simulink model "chap7_1sim"  (R2019a)
settings: Solver=ode45  StartTime=0.0  StopTime=10.0  RelTol=1e-3
settings Model: Creator=smilingfrog  LastModifiedBy=smilingfrog
settings DataIOCC: SaveOutput=off  SignalLogging=off  DSMLogging=off  SaveTime=off  ReturnWorkspaceOutputs=off

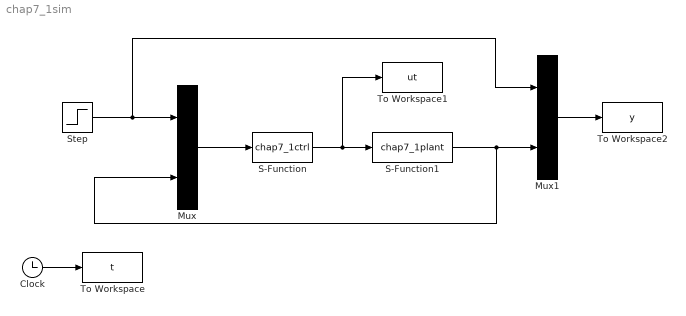
== system chap7_1sim ==
  Clock : Clock
  Mux : Mux  Inputs=2
  Mux1 : Mux  Inputs=2
  S-Function : S-Function  FunctionName=chap7_1ctrl  SFunctionDeploymentMode=off  EnableBusSupport=off
  S-Function1 : S-Function  FunctionName=chap7_1plant  SFunctionDeploymentMode=off  EnableBusSupport=off
  Step : Step  Time=0  SampleTime=0
  To Workspace : ToWorkspace  VariableName=t  SampleTime=-1
  To Workspace1 : ToWorkspace  VariableName=ut  SampleTime=-1
  To Workspace2 : ToWorkspace  VariableName=y  SampleTime=-1
  wires:
  Step/1 -> Mux1/1, Mux/1
  S-Function/1 -> To Workspace1/1, S-Function1/1
  Mux/1 -> S-Function/1
  Clock/1 -> To Workspace/1
  S-Function1/1 -> Mux/2, Mux1/2
  Mux1/1 -> To Workspace2/1
